simulink model "PlantArch"  (R2021b)
settings: Solver=VariableStepAuto  StartTime=0.0  StopTime=10.0  RelTol=1e-3
undefined symbols (not defined in the file or in its folder): N, P
libraries: nesl_utility x17, fl_lib x15, ee_lib x9
settings Model: DataDictionary=ZC_EVPowerSystem.sldd  Creator=ykamatan  LastModifiedBy=ykamatan

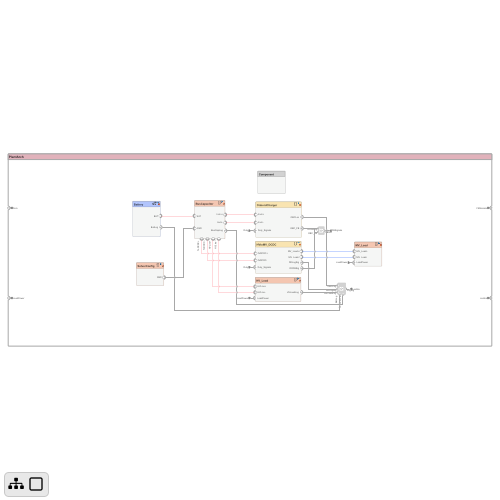
[thumbnail: Simulink's stored preview of the top-level diagram]
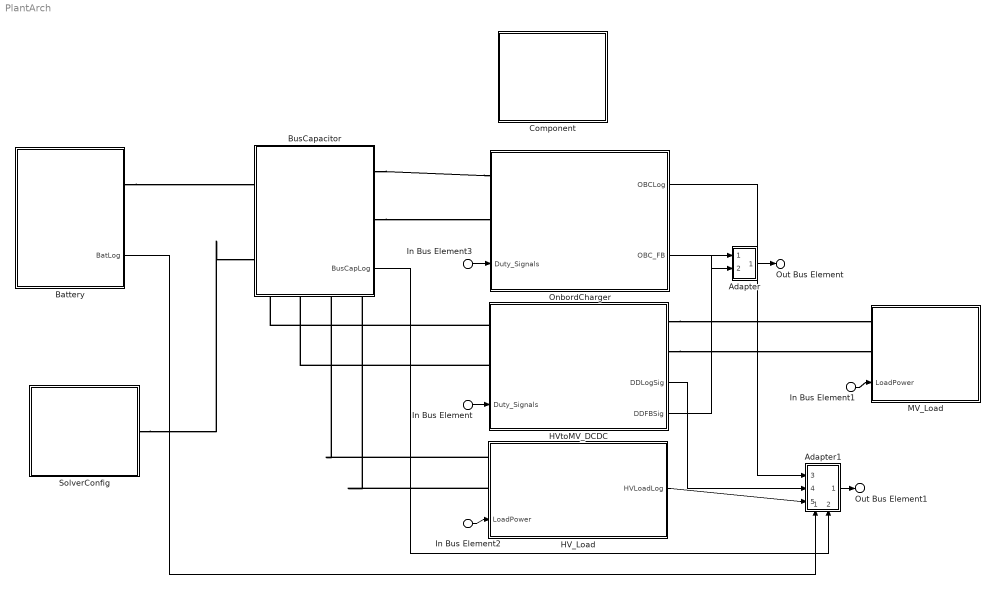
== system PlantArch ==
  In Bus Element : Inport  PortName=Duty
  In Bus Element3 : Inport  PortName=Duty
  In Bus Element1 : Inport  Port=2  PortName=LoadPower
  In Bus Element2 : Inport  Port=2  PortName=LoadPower
  Adapter : Subsystem
      settings: PortSchema="{\"entries\":[{\"content\":{\"margin\":10,\"minimumSpacing\":15,\"sides\":[{\"content\":{\"connectorIds\":[\"In1\",\"In2\"]},\"type\":\"ConnectorPlacement.EquallySpacedRectSide\",\"uuid\":\"68f5454e-c2f0-4736-99c3-02080df13840\"},{\"content\":{\"connectorIds\":[\"Out1\"],\"side\":\"RIGHT\"},\"type\":\"ConnectorPlacement.EquallySpacedRectSide\",\"uuid\":\"5ee879a6-3050-43f8-b648-386fe489b578\"},{\"content\":{\"connectorIds\":[],\"side\":\"TOP\"},\"type\":\"ConnectorPlacement.EquallySpacedRectSide\",\"uuid\":\"ef80faa4-f045-40f6-9eb7-7f3a67b10a8e\"}]},\"type\":\"ConnectorPlacement.EquallySpacedConnector\",\"uuid\":\"bb0e3b0d-aad0-4c98-a3b7-f5aab2b06e29\"}],\"packageUris\":[\"http://schema.mathworks.com/mf0/Connector/R2020b\"],\"version\":\"1.0\"}"
  Adapter1 : Subsystem
      settings: PortSchema="{\"entries\":[{\"content\":{\"margin\":10,\"minimumSpacing\":15,\"sides\":[{\"content\":{\"connectorIds\":[\"In3\",\"In4\",\"In5\"]},\"type\":\"ConnectorPlacement.EquallySpacedRectSide\",\"uuid\":\"68f5454e-c2f0-4736-99c3-02080df13840\"},{\"content\":{\"connectorIds\":[\"Out1\"],\"side\":\"RIGHT\"},\"type\":\"ConnectorPlacement.EquallySpacedRectSide\",\"uuid\":\"5ee879a6-3050-43f8-b648-386fe489b578\"},{\"content\":{\"connectorIds\":[],\"side\":\"TOP\"},\"type\":\"ConnectorPlacement.EquallySpacedRectSide\",\"uuid\":\"ef80faa4-f045-40f6-9eb7-7f3a67b10a8e\"},{\"content\":{\"connectorIds\":[\"In1\",\"In2\"],\"side\":\"BOTTOM\"},\"type\":\"ConnectorPlacement.EquallySpacedRectSide\",\"uuid\":\"e02d8c0b-11c6-4468-90e5-a6f684fa16b6\"}]},\"type\":\"ConnectorPlacement.EquallySpacedConnector\",\"uuid\":\"bb0e3b0d-aad0-4c98-a3b7-f5aab2b06e29\"}],\"packageUris\":[\"http://schema.mathworks.com/mf0/Connector/R2020b\"],\"version\":\"1.0\"}"
  Battery : Subsystem
      settings: PortSchema="{\"entries\":[{\"content\":{\"headerSize\":26,\"margin\":15,\"minimumSpacing\":25,\"sides\":[{\"content\":{\"connectorIds\":[]},\"type\":\"ConnectorPlacement.EquallySpacedRectSide\",\"uuid\":\"bc9bb9ba-2a95-4d32-9fa4-7976113ef647\"},{\"content\":{\"connectorIds\":[\"RConn1\",\"Out1\"],\"side\":\"RIGHT\"},\"type\":\"ConnectorPlacement.EquallySpacedRectSide\",\"uuid\":\"964ff6e2-b516-444b-80c9-2869b54c1800\"},{\"content\":{\"connectorIds\":[],\"side\":\"TOP\"},\"type\":\"ConnectorPlacement.EquallySpacedRectSide\",\"uuid\":\"d01200aa-db6c-474b-a6ec-1bd59e1bf90f\"}]},\"type\":\"ConnectorPlacement.EquallySpacedConnector\",\"uuid\":\"135e4cd7-10c4-47f4-80e9-6ecafc5508de\"}],\"packageUris\":[\"http://schema.mathworks.com/mf0/Connector/R2020b\"],\"version\":\"1.0\"}"
  BusCapacitor : Subsystem
      settings: PortSchema="{\"entries\":[{\"content\":{\"headerSize\":26,\"margin\":15,\"minimumSpacing\":25,\"sides\":[{\"content\":{\"connectorIds\":[\"LConn1\",\"LConn2\"]},\"type\":\"ConnectorPlacement.EquallySpacedRectSide\",\"uuid\":\"bc9bb9ba-2a95-4d32-9fa4-7976113ef647\"},{\"content\":{\"connectorIds\":[\"RConn5\",\"RConn6\",\"Out1\"],\"side\":\"RIGHT\"},\"type\":\"ConnectorPlacement.EquallySpacedRectSide\",\"uuid\":\"964ff6e2-b516-444b-80c9-2869b54c1800\"},{\"content\":{\"connectorIds\":[],\"side\":\"TOP\"},\"type\":\"ConnectorPlacement.EquallySpacedRectSide\",\"uuid\":\"d01200aa-db6c-474b-a6ec-1bd59e1bf90f\"},{\"content\":{\"connectorIds\":[\"RConn1\",\"RConn2\",\"RConn3\",\"RConn4\"],\"side\":\"BOTTOM\"},\"type\":\"ConnectorPlacement.EquallySpacedRectSide\",\"uuid\":\"7b919d1c-288c-41a8-8fd6-bd8ebd8eb2b7\"}]},\"type\":\"ConnectorPlacement.EquallySpacedConnector\",\"uuid\":\"135e4cd7-10c4-47f4-80e9-6ecafc5508de\"}],\"packageUris\":[\"http://schema.mathworks.com/mf0/Connector/R2020b\"],\"version\":\"1.0\"}"
  Component : Subsystem
      settings: PortSchema="{\"entries\":[{\"content\":{\"headerSize\":26,\"margin\":15,\"minimumSpacing\":25,\"sides\":[{\"content\":{\"connectorIds\":[]},\"type\":\"ConnectorPlacement.EquallySpacedRectSide\",\"uuid\":\"03ee5175-8d94-4deb-b18d-1b94bccaf658\"},{\"content\":{\"connectorIds\":[],\"side\":\"RIGHT\"},\"type\":\"ConnectorPlacement.EquallySpacedRectSide\",\"uuid\":\"44db8dae-2982-4fa1-b39b-413b881f7ee2\"},{\"content\":{\"connectorIds\":[],\"side\":\"TOP\"},\"type\":\"ConnectorPlacement.EquallySpacedRectSide\",\"uuid\":\"37e3387e-c8c6-4301-8ebe-99b8cda93072\"}]},\"type\":\"ConnectorPlacement.EquallySpacedConnector\",\"uuid\":\"c90e0097-298e-4f62-a136-d8f6219bd626\"}],\"packageUris\":[\"http://schema.mathworks.com/mf0/Connector/R2020b\"],\"version\":\"1.0\"}"
  HV_Load : Subsystem
      settings: PortSchema="{\"entries\":[{\"content\":{\"headerSize\":26,\"margin\":15,\"minimumSpacing\":25,\"sides\":[{\"content\":{\"connectorIds\":[\"LConn1\",\"LConn2\",\"In1\"]},\"type\":\"ConnectorPlacement.EquallySpacedRectSide\",\"uuid\":\"bc9bb9ba-2a95-4d32-9fa4-7976113ef647\"},{\"content\":{\"connectorIds\":[\"Out1\"],\"side\":\"RIGHT\"},\"type\":\"ConnectorPlacement.EquallySpacedRectSide\",\"uuid\":\"964ff6e2-b516-444b-80c9-2869b54c1800\"},{\"content\":{\"connectorIds\":[],\"side\":\"TOP\"},\"type\":\"ConnectorPlacement.EquallySpacedRectSide\",\"uuid\":\"d01200aa-db6c-474b-a6ec-1bd59e1bf90f\"}]},\"type\":\"ConnectorPlacement.EquallySpacedConnector\",\"uuid\":\"135e4cd7-10c4-47f4-80e9-6ecafc5508de\"}],\"packageUris\":[\"http://schema.mathworks.com/mf0/Connector/R2020b\"],\"version\":\"1.0\"}"
  HVtoMV_DCDC : Subsystem
      settings: PortSchema="{\"entries\":[{\"content\":{\"headerSize\":26,\"margin\":15,\"minimumSpacing\":25,\"sides\":[{\"content\":{\"connectorIds\":[\"LConn1\",\"LConn2\",\"In1\"]},\"type\":\"ConnectorPlacement.EquallySpacedRectSide\",\"uuid\":\"bc9bb9ba-2a95-4d32-9fa4-7976113ef647\"},{\"content\":{\"connectorIds\":[\"RConn1\",\"RConn2\",\"Out1\",\"Out2\"],\"side\":\"RIGHT\"},\"type\":\"ConnectorPlacement.EquallySpacedRectSide\",\"uuid\":\"964ff6e2-b516-444b-80c9-2869b54c1800\"},{\"content\":{\"connectorIds\":[],\"side\":\"TOP\"},\"type\":\"ConnectorPlacement.EquallySpacedRectSide\",\"uuid\":\"d01200aa-db6c-474b-a6ec-1bd59e1bf90f\"}]},\"type\":\"ConnectorPlacement.EquallySpacedConnector\",\"uuid\":\"135e4cd7-10c4-47f4-80e9-6ecafc5508de\"}],\"packageUris\":[\"http://schema.mathworks.com/mf0/Connector/R2020b\"],\"version\":\"1.0\"}"
  MV_Load : Subsystem
      settings: PortSchema="{\"entries\":[{\"content\":{\"headerSize\":26,\"margin\":15,\"minimumSpacing\":25,\"sides\":[{\"content\":{\"connectorIds\":[\"LConn1\",\"LConn2\",\"In1\"]},\"type\":\"ConnectorPlacement.EquallySpacedRectSide\",\"uuid\":\"bc9bb9ba-2a95-4d32-9fa4-7976113ef647\"},{\"content\":{\"connectorIds\":[],\"side\":\"RIGHT\"},\"type\":\"ConnectorPlacement.EquallySpacedRectSide\",\"uuid\":\"964ff6e2-b516-444b-80c9-2869b54c1800\"},{\"content\":{\"connectorIds\":[],\"side\":\"TOP\"},\"type\":\"ConnectorPlacement.EquallySpacedRectSide\",\"uuid\":\"d01200aa-db6c-474b-a6ec-1bd59e1bf90f\"}]},\"type\":\"ConnectorPlacement.EquallySpacedConnector\",\"uuid\":\"135e4cd7-10c4-47f4-80e9-6ecafc5508de\"}],\"packageUris\":[\"http://schema.mathworks.com/mf0/Connector/R2020b\"],\"version\":\"1.0\"}"
  OnbordCharger : Subsystem
      settings: PortSchema="{\"entries\":[{\"content\":{\"headerSize\":26,\"margin\":15,\"minimumSpacing\":25,\"sides\":[{\"content\":{\"connectorIds\":[\"LConn1\",\"LConn2\",\"In1\"]},\"type\":\"ConnectorPlacement.EquallySpacedRectSide\",\"uuid\":\"bc9bb9ba-2a95-4d32-9fa4-7976113ef647\"},{\"content\":{\"connectorIds\":[\"Out1\",\"Out2\"],\"side\":\"RIGHT\"},\"type\":\"ConnectorPlacement.EquallySpacedRectSide\",\"uuid\":\"964ff6e2-b516-444b-80c9-2869b54c1800\"},{\"content\":{\"connectorIds\":[],\"side\":\"TOP\"},\"type\":\"ConnectorPlacement.EquallySpacedRectSide\",\"uuid\":\"d01200aa-db6c-474b-a6ec-1bd59e1bf90f\"}]},\"type\":\"ConnectorPlacement.EquallySpacedConnector\",\"uuid\":\"135e4cd7-10c4-47f4-80e9-6ecafc5508de\"}],\"packageUris\":[\"http://schema.mathworks.com/mf0/Connector/R2020b\"],\"version\":\"1.0\"}"
  SolverConfig : Subsystem
      settings: PortSchema="{\"entries\":[{\"content\":{\"headerSize\":26,\"margin\":15,\"minimumSpacing\":25,\"sides\":[{\"content\":{\"connectorIds\":[]},\"type\":\"ConnectorPlacement.EquallySpacedRectSide\",\"uuid\":\"bc9bb9ba-2a95-4d32-9fa4-7976113ef647\"},{\"content\":{\"connectorIds\":[\"RConn1\"],\"side\":\"RIGHT\"},\"type\":\"ConnectorPlacement.EquallySpacedRectSide\",\"uuid\":\"964ff6e2-b516-444b-80c9-2869b54c1800\"},{\"content\":{\"connectorIds\":[],\"side\":\"TOP\"},\"type\":\"ConnectorPlacement.EquallySpacedRectSide\",\"uuid\":\"d01200aa-db6c-474b-a6ec-1bd59e1bf90f\"}]},\"type\":\"ConnectorPlacement.EquallySpacedConnector\",\"uuid\":\"135e4cd7-10c4-47f4-80e9-6ecafc5508de\"}],\"packageUris\":[\"http://schema.mathworks.com/mf0/Connector/R2020b\"],\"version\":\"1.0\"}"
  Out Bus Element : Outport  PortName=FBSignals
  Out Bus Element1 : Outport  Port=2  PortName=LogSig
  wires:
  In Bus Element1/1 -> MV_Load/1(LoadPower)
  In Bus Element/1 -> HVtoMV_DCDC/1(Duty_Signals)
  In Bus Element3/1 -> OnbordCharger/1(Duty_Signals)
  Adapter/1(FBSig) -> Out Bus Element/1
  Adapter1/1(LogSig) -> Out Bus Element1/1
  In Bus Element2/1 -> HV_Load/1(LoadPower)
  Battery/1(BatLog) -> Adapter1/1(BatLog)
  BusCapacitor/1(BusCapLog) -> Adapter1/2(BusCapLog)
  OnbordCharger/1(OBCLog) -> Adapter1/3(OBCLog)
  HVtoMV_DCDC/1(DDLogSig) -> Adapter1/4(DDLogSig)
  HV_Load/1(HVLoadLog) -> Adapter1/5(HVLoadLog)
  HVtoMV_DCDC/2(DDFBSig) -> Adapter/1(DDFBSig)
  OnbordCharger/2(OBC_FB) -> Adapter/2(OBC_FB)
  connections:
  HVtoMV_DCDC/RConn1 -- MV_Load/LConn1
  HVtoMV_DCDC/RConn2 -- MV_Load/LConn2
  HV_Load/LConn1 -- BusCapacitor/RConn3
  HV_Load/LConn2 -- BusCapacitor/RConn4
  HVtoMV_DCDC/LConn1 -- BusCapacitor/RConn1
  HVtoMV_DCDC/LConn2 -- BusCapacitor/RConn2
  BusCapacitor/RConn5 -- OnbordCharger/LConn1
  BusCapacitor/RConn6 -- OnbordCharger/LConn2
  SolverConfig/RConn1 -- BusCapacitor/LConn2
  Battery/RConn1 -- BusCapacitor/LConn1

== system PlantArch/Adapter ==
  Bus Element In2 : Inport  PortName=DDFBSig
  Bus Element In1 : Inport  Port=2  PortName=OBC_FB
  Out Bus Element : Outport  PortName=FBSig  Element=DD_FBSig
  BEP : Outport  PortName=FBSig  Element=PFC_FBSig
  wires:
  Bus Element In2/1 -> Out Bus Element/1
  Bus Element In1/1 -> BEP/1

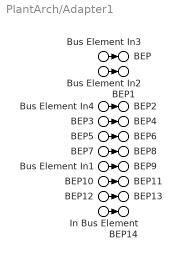
== system PlantArch/Adapter1 ==
  Bus Element In4 : Inport  PortName=BatLog  Element=iDC
  Bus Element In3 : Inport  Port=2  PortName=BusCapLog  Element=vDC
  Bus Element In2 : Inport  Port=3  PortName=OBCLog  Element=iL
  BEP3 : Inport  Port=3  PortName=OBCLog  Element=iDCInv
  BEP5 : Inport  Port=3  PortName=OBCLog  Element=vInv
  BEP7 : Inport  Port=3  PortName=OBCLog  Element=vs
  Bus Element In1 : Inport  Port=4  PortName=DDLogSig  Element=iLoad48V
  BEP10 : Inport  Port=4  PortName=DDLogSig  Element=iDC48VBass
  BEP12 : Inport  Port=4  PortName=DDLogSig  Element=v48VBass
  In Bus Element : Inport  Port=5  PortName=HVLoadLog  Element=iDC400VBass
  BEP1 : Outport  PortName=LogSig  Element=iL
  BEP2 : Outport  PortName=LogSig  Element=iDC
  BEP4 : Outport  PortName=LogSig  Element=iDCInv
  BEP9 : Outport  PortName=LogSig  Element=iLoad48V
  BEP11 : Outport  PortName=LogSig  Element=iDC48VBass
  BEP14 : Outport  PortName=LogSig  Element=iDC400VBass
  BEP : Outport  PortName=LogSig  Element=vDC
  BEP6 : Outport  PortName=LogSig  Element=vInv
  BEP8 : Outport  PortName=LogSig  Element=vs
  BEP13 : Outport  PortName=LogSig  Element=v48VBass
  wires:
  Bus Element In4/1 -> BEP2/1
  Bus Element In3/1 -> BEP/1
  Bus Element In2/1 -> BEP1/1
  BEP3/1 -> BEP4/1
  BEP5/1 -> BEP6/1
  BEP7/1 -> BEP8/1
  Bus Element In1/1 -> BEP9/1
  BEP10/1 -> BEP11/1
  BEP12/1 -> BEP13/1
  In Bus Element/1 -> BEP14/1

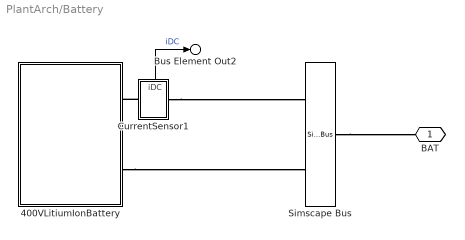
== system PlantArch/Battery ==
  400VLitiumIonBattery : Subsystem
  CurrentSensor1 : Subsystem
      settings: PortSchema="{\"entries\":[{\"content\":{\"sides\":[{\"content\":{\"connectorIds\":[\"LConn1\"]},\"type\":\"ConnectorPlacement.EquallySpacedRectSide\",\"uuid\":\"7286f59e-cee0-499d-832c-cf6f33a1b017\"},{\"content\":{\"connectorIds\":[\"RConn1\"],\"side\":\"RIGHT\"},\"type\":\"ConnectorPlacement.EquallySpacedRectSide\",\"uuid\":\"6a983281-a6bc-4a57-a5ba-c4da9a8828f4\"},{\"content\":{\"connectorIds\":[\"Out1\"],\"side\":\"TOP\"},\"type\":\"ConnectorPlacement.EquallySpacedRectSide\",\"uuid\":\"6969f7e7-2dce-4d64-b6f6-e92ef9035b1a\"}]},\"type\":\"ConnectorPlacement.EquallySpacedConnector\",\"uuid\":\"05fc616a-5402-4b75-b59e-8cf259d71f3d\"}],\"packageUris\":[\"http://schema.mathworks.com/mf0/Connector/R2020b\"],\"version\":\"1.0\"}"
  Simscape Bus : SimscapeBus  HierarchyStrings=P;N  ConnectionType=Bus: HV_PowerLine
  BAT : PMIOPort  Side=Right  ConnectionType=Bus: HV_PowerLine
  Bus Element Out2 : Outport  PortName=BatLog  Element=iDC
  wires:
  CurrentSensor1/1(iDC) -> Bus Element Out2/1  "iDC"
  connections:
  CurrentSensor1/LConn1 -- 400VLitiumIonBattery/RConn1
  CurrentSensor1/RConn1 -- Simscape Bus/LConn1
  400VLitiumIonBattery/RConn2 -- Simscape Bus/LConn2
  Simscape Bus/RConn1 -- BAT/RConn1

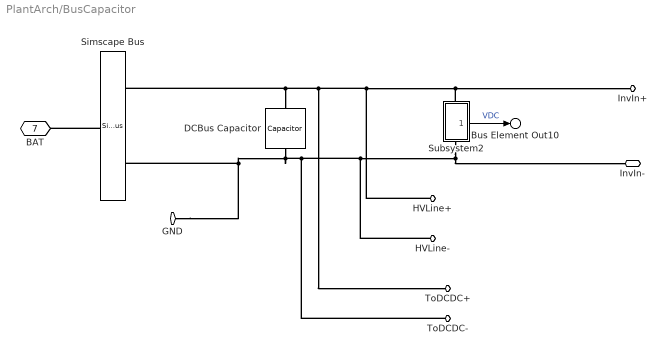
== system PlantArch/BusCapacitor ==
  DCBus Capacitor : ee_lib/Passive/Capacitor  cap_option=0  c=1000e-6 F  Cvec=[1e-05, 1e-06] F  Vvec=[0, 10] V  CV_table_symmetry=1  f_vec=[1, 10] kHz  DFext_vec=[.8, 1.2]  C_tol=5  enable_C_tol=0  tol_distribution=1  nSigma=4  r=1e-6 Ohm  g=0 1/Ohm  averaging_period=0 s  enable_operating_limits=0  operating_limit_action=2  max_working_voltage_range=[-25, 25] V  power_rating=1 W  enable_faults=0  fault_action=1  Cscale_faulted=100  R_faulted=1e-3 Ohm  G_faulted=0 1/Ohm  tau_fault=1e-3 s  enable_temporal_fault=0  t_fault=1 s  enable_behavioral_fault=0  max_permissible_voltage_range=[-100, 100] V  t_fail_on_voltage=1 s  i_specify=off  i_priority=None  i=0 A  i_nominal_specify=off  i_nominal_unit=A  i_nominal_value=1  v_specify=off  v_priority=None  v=400 V  v_nominal_specify=off  v_nominal_unit=V  v_nominal_value=1  vc_specify=on  vc_priority=High  vc=400 V  vc_nominal_specify=off  vc_nominal_unit=V  vc_nominal_value=1
  Simscape Bus : SimscapeBus  HierarchyStrings=P;N  ConnectionType=Bus: HV_PowerLine
  Subsystem2 : Subsystem
      settings: PortSchema="{\"entries\":[{\"content\":{\"sides\":[{\"content\":{\"connectorIds\":[]},\"type\":\"ConnectorPlacement.EquallySpacedRectSide\",\"uuid\":\"7286f59e-cee0-499d-832c-cf6f33a1b017\"},{\"content\":{\"connectorIds\":[\"Out1\"],\"side\":\"RIGHT\"},\"type\":\"ConnectorPlacement.EquallySpacedRectSide\",\"uuid\":\"6a983281-a6bc-4a57-a5ba-c4da9a8828f4\"},{\"content\":{\"connectorIds\":[\"LConn1\"],\"side\":\"TOP\"},\"type\":\"ConnectorPlacement.EquallySpacedRectSide\",\"uuid\":\"6969f7e7-2dce-4d64-b6f6-e92ef9035b1a\"},{\"content\":{\"connectorIds\":[\"RConn1\"],\"side\":\"BOTTOM\"},\"type\":\"ConnectorPlacement.EquallySpacedRectSide\",\"uuid\":\"8f7d22cd-967a-487e-912d-7270502758f1\"}]},\"type\":\"ConnectorPlacement.EquallySpacedConnector\",\"uuid\":\"05fc616a-5402-4b75-b59e-8cf259d71f3d\"}],\"packageUris\":[\"http://schema.mathworks.com/mf0/Connector/R2020b\"],\"version\":\"1.0\"}"
  ToDCDC+ : PMIOPort  Side=Right
  ToDCDC- : PMIOPort  Port=2  Side=Right
  HVLine+ : PMIOPort  Port=3  Side=Right
  HVLine- : PMIOPort  Port=4  Side=Right
  InvIn+ : PMIOPort  Port=5  Side=Right
  InvIn- : PMIOPort  Port=6  Side=Right
  BAT : PMIOPort  Port=7  Side=Left  ConnectionType=Bus: HV_PowerLine
  GND : PMIOPort  Port=8  Side=Left
  Bus Element Out10 : Outport  PortName=BusCapLog  Element=vDC
  wires:
  Subsystem2/1(Vdc) -> Bus Element Out10/1  "VDC"
  connections:
  DCBus Capacitor/RConn1 -- GND/RConn1 -- Simscape Bus/LConn2 -- HVLine-/RConn1 -- InvIn-/RConn1 -- Subsystem2/RConn1 -- ToDCDC-/RConn1
  HVLine+/RConn1 -- InvIn+/RConn1 -- Subsystem2/LConn1 -- ToDCDC+/RConn1 -- DCBus Capacitor/LConn1 -- Simscape Bus/LConn1
  Simscape Bus/RConn1 -- BAT/RConn1

== system PlantArch/Component ==

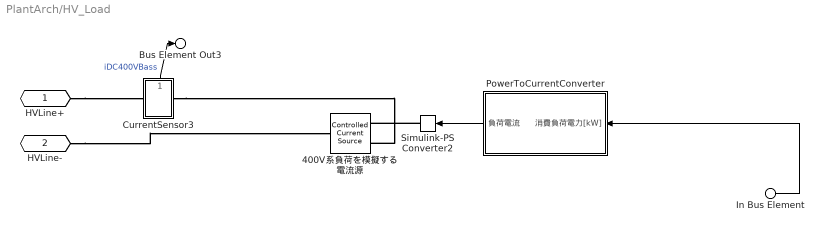
== system PlantArch/HV_Load ==
  In Bus Element : Inport  PortName=LoadPower  Element=Load400V
  400V系負荷を模擬する 電流源 : fl_lib/Electrical/Electrical Sources/Controlled Current Source
  CurrentSensor3 : Subsystem
      settings: PortSchema="{\"entries\":[{\"content\":{\"sides\":[{\"content\":{\"connectorIds\":[\"LConn1\"]},\"type\":\"ConnectorPlacement.EquallySpacedRectSide\",\"uuid\":\"7286f59e-cee0-499d-832c-cf6f33a1b017\"},{\"content\":{\"connectorIds\":[\"RConn1\"],\"side\":\"RIGHT\"},\"type\":\"ConnectorPlacement.EquallySpacedRectSide\",\"uuid\":\"6a983281-a6bc-4a57-a5ba-c4da9a8828f4\"},{\"content\":{\"connectorIds\":[\"Out1\"],\"side\":\"TOP\"},\"type\":\"ConnectorPlacement.EquallySpacedRectSide\",\"uuid\":\"6969f7e7-2dce-4d64-b6f6-e92ef9035b1a\"}]},\"type\":\"ConnectorPlacement.EquallySpacedConnector\",\"uuid\":\"05fc616a-5402-4b75-b59e-8cf259d71f3d\"}],\"packageUris\":[\"http://schema.mathworks.com/mf0/Connector/R2020b\"],\"version\":\"1.0\"}"
  PowerToCurrentConverter : Subsystem
  Simulink-PS Converter2 : nesl_utility/Simulink-PS Converter  PhysicalDomain=network_engine_domain  SubClassName=ps_input  LeftPortType=input  RightPortType=output  PseudoPeriodic=off  Frequencies=[]  NoiseDistribution=none  NoiseParameters=[]  Unit=1  AffineConversion=off  FilteringAndDerivatives=provide  SimscapeFilterOrder=1  InputFilterTimeConstant=0.001  UdotUserProvided=0
      settings: SourceProductBaseCode=PW,SS
  HVLine+ : PMIOPort  Side=Left
  HVLine- : PMIOPort  Port=2  Side=Left
  Bus Element Out3 : Outport  PortName=HVLoadLog  Element=iDC400VBass
  wires:
  CurrentSensor3/1(iDC400VBass) -> Bus Element Out3/1  "iDC400VBass"
  PowerToCurrentConverter/1(負荷電流) -> Simulink-PS Converter2/1
  In Bus Element/1 -> PowerToCurrentConverter/1(消費負荷電力[kW])
  connections:
  Simulink-PS Converter2/RConn1 -- 400V系負荷を模擬する 電流源/RConn1
  CurrentSensor3/RConn1 -- 400V系負荷を模擬する 電流源/RConn2
  HVLine+/RConn1 -- CurrentSensor3/LConn1
  HVLine-/RConn1 -- 400V系負荷を模擬する 電流源/LConn1

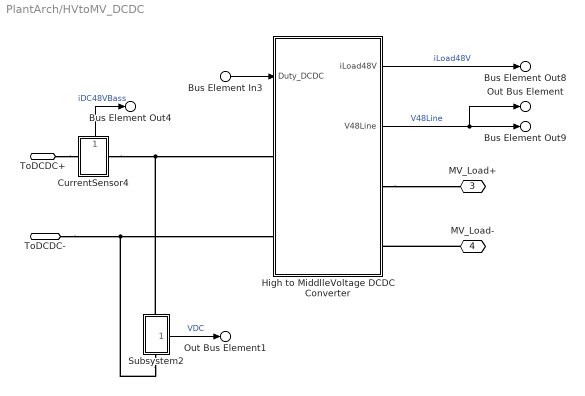
== system PlantArch/HVtoMV_DCDC ==
  Bus Element In3 : Inport  PortName=Duty_Signals  Element=DD48v_Duty
  CurrentSensor4 : Subsystem
      settings: PortSchema="{\"entries\":[{\"content\":{\"sides\":[{\"content\":{\"connectorIds\":[\"LConn1\"]},\"type\":\"ConnectorPlacement.EquallySpacedRectSide\",\"uuid\":\"7286f59e-cee0-499d-832c-cf6f33a1b017\"},{\"content\":{\"connectorIds\":[\"RConn1\"],\"side\":\"RIGHT\"},\"type\":\"ConnectorPlacement.EquallySpacedRectSide\",\"uuid\":\"6a983281-a6bc-4a57-a5ba-c4da9a8828f4\"},{\"content\":{\"connectorIds\":[\"Out1\"],\"side\":\"TOP\"},\"type\":\"ConnectorPlacement.EquallySpacedRectSide\",\"uuid\":\"6969f7e7-2dce-4d64-b6f6-e92ef9035b1a\"}]},\"type\":\"ConnectorPlacement.EquallySpacedConnector\",\"uuid\":\"05fc616a-5402-4b75-b59e-8cf259d71f3d\"}],\"packageUris\":[\"http://schema.mathworks.com/mf0/Connector/R2020b\"],\"version\":\"1.0\"}"
  High to MiddlleVoltage DCDC Converter : Subsystem
  Subsystem2 : Subsystem
      settings: PortSchema="{\"entries\":[{\"content\":{\"sides\":[{\"content\":{\"connectorIds\":[]},\"type\":\"ConnectorPlacement.EquallySpacedRectSide\",\"uuid\":\"7286f59e-cee0-499d-832c-cf6f33a1b017\"},{\"content\":{\"connectorIds\":[\"Out1\"],\"side\":\"RIGHT\"},\"type\":\"ConnectorPlacement.EquallySpacedRectSide\",\"uuid\":\"6a983281-a6bc-4a57-a5ba-c4da9a8828f4\"},{\"content\":{\"connectorIds\":[\"LConn1\"],\"side\":\"TOP\"},\"type\":\"ConnectorPlacement.EquallySpacedRectSide\",\"uuid\":\"6969f7e7-2dce-4d64-b6f6-e92ef9035b1a\"},{\"content\":{\"connectorIds\":[\"RConn1\"],\"side\":\"BOTTOM\"},\"type\":\"ConnectorPlacement.EquallySpacedRectSide\",\"uuid\":\"8f7d22cd-967a-487e-912d-7270502758f1\"}]},\"type\":\"ConnectorPlacement.EquallySpacedConnector\",\"uuid\":\"05fc616a-5402-4b75-b59e-8cf259d71f3d\"}],\"packageUris\":[\"http://schema.mathworks.com/mf0/Connector/R2020b\"],\"version\":\"1.0\"}"
  ToDCDC+ : PMIOPort  Side=Left
  ToDCDC- : PMIOPort  Port=2  Side=Left
  MV_Load+ : PMIOPort  Port=3  Side=Right
  MV_Load- : PMIOPort  Port=4  Side=Right
  Bus Element Out8 : Outport  PortName=DDLogSig  Element=iLoad48V
  Bus Element Out4 : Outport  PortName=DDLogSig  Element=iDC48VBass
  Bus Element Out9 : Outport  PortName=DDLogSig  Element=v48VBass
  Out Bus Element : Outport  Port=2  PortName=DDFBSig  Element=vout
  Out Bus Element1 : Outport  Port=2  PortName=DDFBSig  Element=vin
  wires:
  CurrentSensor4/1(iDC48VBass) -> Bus Element Out4/1  "iDC48VBass"
  Bus Element In3/1 -> High to MiddlleVoltage DCDC Converter/1(Duty_DCDC)
  High to MiddlleVoltage DCDC Converter/2(V48Line) -> Out Bus Element/1, Bus Element Out9/1  "V48Line"
  High to MiddlleVoltage DCDC Converter/1(iLoad48V) -> Bus Element Out8/1  "iLoad48V"
  Subsystem2/1(Vdc) -> Out Bus Element1/1  "VDC"
  connections:
  CurrentSensor4/RConn1 -- Subsystem2/LConn1 -- High to MiddlleVoltage DCDC Converter/LConn1
  High to MiddlleVoltage DCDC Converter/RConn1 -- MV_Load+/RConn1
  MV_Load-/RConn1 -- High to MiddlleVoltage DCDC Converter/RConn2
  ToDCDC+/RConn1 -- CurrentSensor4/LConn1
  ToDCDC-/RConn1 -- Subsystem2/RConn1 -- High to MiddlleVoltage DCDC Converter/LConn2

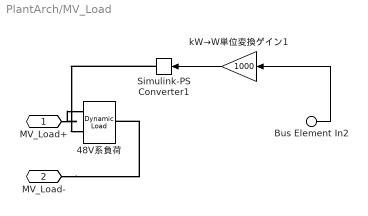
== system PlantArch/MV_Load ==
  Bus Element In2 : Inport  PortName=LoadPower  Element=Load48V
  48V系負荷 : ee_lib/Passive/Dynamic Load  load_type=ee.enum.dc_ac.dc  min_supply_voltage=38 V  pow_min=1e-3 W  G_reverse=1e-6 S  deltaV=1e-3 V  f0=60 Hz  Vrms_min=200 V  Pmin=1e-3 W  enable_fault=simscape.enum.onoff.off  fault_action=simscape.enum.assert.action.none  t_fault=1 s  open_conductance=1e-4 S
      settings: SourceProductBaseCode=PS  InternalSimscapePortConfiguration="{\"Bottom\":[],\"Left\":[{\"id\":\"p\",\"label\":\"+\",\"type\":\"foundation.electrical.electrical\"}],\"Right\":[{\"id\":\"n\",\"label\":\"-\",\"type\":\"foundation.electrical.electrical\"}],\"Top\":[{\"id\":\"P\",\"label\":\"P\",\"type\":\"input\"}]}"
  Simulink-PS Converter1 : nesl_utility/Simulink-PS Converter  PhysicalDomain=network_engine_domain  SubClassName=ps_input  LeftPortType=input  RightPortType=output  PseudoPeriodic=off  Frequencies=[]  NoiseDistribution=none  NoiseParameters=[]  Unit=1  AffineConversion=off  FilteringAndDerivatives=provide  SimscapeFilterOrder=1  InputFilterTimeConstant=0.001  UdotUserProvided=0
      settings: SourceProductBaseCode=PW,SS
  kW→W単位変換ゲイン1 : Gain  Gain=1000
  MV_Load+ : PMIOPort  Side=Left
  MV_Load- : PMIOPort  Port=2  Side=Left
  wires:
  kW→W単位変換ゲイン1/1 -> Simulink-PS Converter1/1
  Bus Element In2/1 -> kW→W単位変換ゲイン1/1
  connections:
  Simulink-PS Converter1/RConn1 -- 48V系負荷/LConn2
  MV_Load-/RConn1 -- 48V系負荷/RConn1
  MV_Load+/RConn1 -- 48V系負荷/LConn1

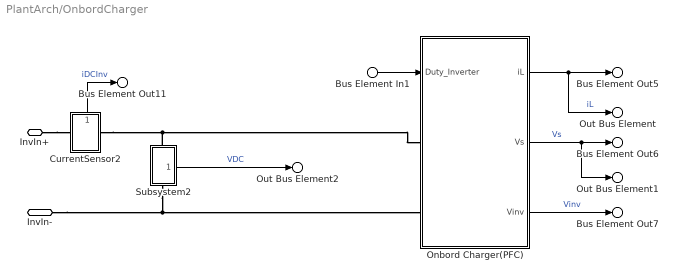
== system PlantArch/OnbordCharger ==
  Bus Element In1 : Inport  PortName=Duty_Signals  Element=PFC_Duty
  CurrentSensor2 : Subsystem
      settings: PortSchema="{\"entries\":[{\"content\":{\"sides\":[{\"content\":{\"connectorIds\":[\"LConn1\"]},\"type\":\"ConnectorPlacement.EquallySpacedRectSide\",\"uuid\":\"7286f59e-cee0-499d-832c-cf6f33a1b017\"},{\"content\":{\"connectorIds\":[\"RConn1\"],\"side\":\"RIGHT\"},\"type\":\"ConnectorPlacement.EquallySpacedRectSide\",\"uuid\":\"6a983281-a6bc-4a57-a5ba-c4da9a8828f4\"},{\"content\":{\"connectorIds\":[\"Out1\"],\"side\":\"TOP\"},\"type\":\"ConnectorPlacement.EquallySpacedRectSide\",\"uuid\":\"6969f7e7-2dce-4d64-b6f6-e92ef9035b1a\"}]},\"type\":\"ConnectorPlacement.EquallySpacedConnector\",\"uuid\":\"05fc616a-5402-4b75-b59e-8cf259d71f3d\"}],\"packageUris\":[\"http://schema.mathworks.com/mf0/Connector/R2020b\"],\"version\":\"1.0\"}"
  Onbord Charger(PFC) : Subsystem
  Subsystem2 : Subsystem
      settings: PortSchema="{\"entries\":[{\"content\":{\"sides\":[{\"content\":{\"connectorIds\":[]},\"type\":\"ConnectorPlacement.EquallySpacedRectSide\",\"uuid\":\"7286f59e-cee0-499d-832c-cf6f33a1b017\"},{\"content\":{\"connectorIds\":[\"Out1\"],\"side\":\"RIGHT\"},\"type\":\"ConnectorPlacement.EquallySpacedRectSide\",\"uuid\":\"6a983281-a6bc-4a57-a5ba-c4da9a8828f4\"},{\"content\":{\"connectorIds\":[\"LConn1\"],\"side\":\"TOP\"},\"type\":\"ConnectorPlacement.EquallySpacedRectSide\",\"uuid\":\"6969f7e7-2dce-4d64-b6f6-e92ef9035b1a\"},{\"content\":{\"connectorIds\":[\"RConn1\"],\"side\":\"BOTTOM\"},\"type\":\"ConnectorPlacement.EquallySpacedRectSide\",\"uuid\":\"8f7d22cd-967a-487e-912d-7270502758f1\"}]},\"type\":\"ConnectorPlacement.EquallySpacedConnector\",\"uuid\":\"05fc616a-5402-4b75-b59e-8cf259d71f3d\"}],\"packageUris\":[\"http://schema.mathworks.com/mf0/Connector/R2020b\"],\"version\":\"1.0\"}"
  InvIn+ : PMIOPort  Side=Left
  InvIn- : PMIOPort  Port=2  Side=Left
  Bus Element Out5 : Outport  PortName=OBCLog  Element=iL
  Bus Element Out11 : Outport  PortName=OBCLog  Element=iDCInv
  Bus Element Out7 : Outport  PortName=OBCLog  Element=vInv
  Bus Element Out6 : Outport  PortName=OBCLog  Element=vs
  Out Bus Element1 : Outport  Port=2  PortName=OBC_FB  Element=vs
  Out Bus Element2 : Outport  Port=2  PortName=OBC_FB  Element=vdc
  Out Bus Element : Outport  Port=2  PortName=OBC_FB  Element=iL
  wires:
  Onbord Charger(PFC)/2(Vs) -> Out Bus Element1/1, Bus Element Out6/1  "Vs"
  Onbord Charger(PFC)/3(Vinv) -> Bus Element Out7/1  "Vinv"
  Onbord Charger(PFC)/1(iL) -> Out Bus Element/1, Bus Element Out5/1  "iL"
  Bus Element In1/1 -> Onbord Charger(PFC)/1(Duty_Inverter)
  CurrentSensor2/1(iDCInv) -> Bus Element Out11/1  "iDCInv"
  Subsystem2/1(Vdc) -> Out Bus Element2/1  "VDC"
  connections:
  CurrentSensor2/RConn1 -- Subsystem2/LConn1 -- Onbord Charger(PFC)/LConn1
  InvIn-/RConn1 -- Subsystem2/RConn1 -- Onbord Charger(PFC)/LConn2
  InvIn+/RConn1 -- CurrentSensor2/LConn1

== system PlantArch/SolverConfig ==
  Electrical Reference : fl_lib/Electrical/Electrical Elements/Electrical Reference
  Solver Configuration : nesl_utility/Solver Configuration  PhysicalDomain=network_engine_domain  SubClassName=solver  LeftPortType=input  RightPortType=generic  Tones=[]  Harmonics=[]  SimulateNoise=off  Profile=off  UseLocalSampling=off  EnableSwitchedLinearOptims=on  FrequencyDomain=off  UseCCode=off  RelTol=0.001  AbsTol=1e-06  MinStep=1e-09  ToWorkspace=off  RevertToSquareIcSolve=off  NumHomotopyIterations=100  PhasorMode=off  PhasorModeNumHarmonics=1  DoDC=off  ResidualTolerance=1e-09  UseLocalSolver=off  LocalSolverChoice=NE_BACKWARD_EULER_ADVANCER  LocalSolverSampleTime=0.001  DoFixedCost=off  MaxNonlinIter=3  MaxModeIter=2  ComputeImpulses=off  ImpulseIterations=2  LinearAlgebra=auto  EquationFormulation=NE_TIME_EF  DelaysMemoryBudget=1024  AutomaticFiltering=on  FilteringTimeConstant=0.001  PartitionStorageMethod=AS_NEEDED  PartitionMemoryBudget=1024  PartitionMethod=ROBUST
      settings: SourceProductBaseCode=PW,SS
  GND : PMIOPort  Side=Right
  connections:
  Electrical Reference/LConn1 -- GND/RConn1 -- Solver Configuration/RConn1

== system PlantArch/Battery/400VLitiumIonBattery ==
  400V 理想特性蓄電池 : ee_lib/Sources/Battery  Vnom=400 V  prm_dir=1  R1_dis=2 Ohm  R1_ch=2 Ohm  R1=1 Ohm  prm_AH=2  AH=0.5 hr*A  V1=380 V  AH1=0.25 hr*A  prm_R2=1  R2=2000 Ohm  prm_dyn=2  Rp1=0.05 Ohm  tau1=30 s  Rp2=0.005 Ohm  tau2=30 s  Rp3=0.005 Ohm  tau3=30 s  Rp4=0.005 Ohm  tau4=30 s  Rp5=0.005 Ohm  tau5=30 s  prm_fade=1  N_fade=100  AH_fade=45 hr*A  R1_fade=2.02 Ohm  R1_ch_fade=2.02 Ohm  V1_fade=10.35 V  prm_age=1  prm_age_OCV=1  OCV_age=0.9  SOC_age=60  delta_time_age_vec=[0] d  temperature_age_vec=[273] K  OCV_scaling_age=2.2134e6  OCV_offset_age=1.632e6  temp_exp_age=0.515833569 V  t_exp_age=0.75  i_specify=off  i_priority=None  i=0 A  i_nominal_specify=off  i_nominal_unit=A  i_nominal_value=1  v_specify=off  v_priority=None  v=0 V  v_nominal_specify=off  v_nominal_unit=V  v_nominal_value=1  charge_specify=on  charge_priority=High  charge=0.25 hr*A  charge_nominal_specify=off  charge_nominal_unit=hr*A  charge_nominal_value=1  num_cycles_specify=off  num_cycles_priority=High  num_cycles=0  num_cycles_nominal_specify=off  num_cycles_nominal_unit=1  num_cycles_nominal_value=1  Tmeas=298.15 K  Tmeas_age=298.15 K  Vnom_T2=12 V  R1_T2=2.2 Ohm  R1_T2_dis=2.2 Ohm  R1_T2_ch=2.2 Ohm  V1_T2=11.4 V  R2_T2=2200 Ohm  Rp1_T2=0.005 Ohm  tau1_T2=30 s  Rp2_T2=0.005 Ohm  tau2_T2=30 s  Rp3_T2=0.005 Ohm  tau3_T2=30 s  Rp4_T2=0.005 Ohm  tau4_T2=30 s  Rp5_T2=0.005 Ohm  tau5_T2=30 s  Tmeas2=273.15 K  thermal_mass=30000 J/K  temperature_specify=off  temperature_priority=High  temperature=298.15 K  temperature_nominal_specify=off  temperature_nominal_unit=K  temperature_nominal_value=1
  Bat+ : PMIOPort  Side=Right
  Bat- : PMIOPort  Port=2  Side=Right
  connections:
  400V 理想特性蓄電池/RConn1 -- Bat-/RConn1
  Bat+/RConn1 -- 400V 理想特性蓄電池/LConn1

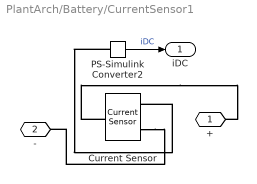
== system PlantArch/Battery/CurrentSensor1 ==
  Current Sensor : fl_lib/Electrical/Electrical Sensors/Current Sensor
  PS-Simulink Converter2 : nesl_utility/PS-Simulink Converter  PhysicalDomain=network_engine_domain  SubClassName=ps_output  LeftPortType=input  RightPortType=output  PseudoPeriodic=off  Frequencies=[]  Unit=inherit  AffineConversion=off
      settings: SourceProductBaseCode=PW,SS
  + : PMIOPort  Side=Left
  - : PMIOPort  Port=2  Side=Right
  iDC : Outport
  wires:
  PS-Simulink Converter2/1 -> iDC/1  "iDC"
  connections:
  Current Sensor/RConn2 -- -/RConn1
  PS-Simulink Converter2/LConn1 -- Current Sensor/RConn1
  Current Sensor/LConn1 -- +/RConn1

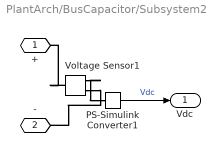
== system PlantArch/BusCapacitor/Subsystem2 ==
  PS-Simulink Converter1 : nesl_utility/PS-Simulink Converter  PhysicalDomain=network_engine_domain  SubClassName=ps_output  LeftPortType=input  RightPortType=output  PseudoPeriodic=off  Frequencies=[]  Unit=inherit  AffineConversion=off
      settings: SourceProductBaseCode=PW,SS
  Voltage Sensor1 : fl_lib/Electrical/Electrical Sensors/Voltage Sensor
  + : PMIOPort  Side=Left
  - : PMIOPort  Port=2  Side=Right
  Vdc : Outport
  wires:
  PS-Simulink Converter1/1 -> Vdc/1  "Vdc"
  connections:
  Voltage Sensor1/RConn2 -- -/RConn1
  Voltage Sensor1/LConn1 -- +/RConn1
  Voltage Sensor1/RConn1 -- PS-Simulink Converter1/LConn1

== system PlantArch/HV_Load/CurrentSensor3 ==
  Current Sensor : fl_lib/Electrical/Electrical Sensors/Current Sensor
  PS-Simulink Converter2 : nesl_utility/PS-Simulink Converter  PhysicalDomain=network_engine_domain  SubClassName=ps_output  LeftPortType=input  RightPortType=output  PseudoPeriodic=off  Frequencies=[]  Unit=inherit  AffineConversion=off
      settings: SourceProductBaseCode=PW,SS
  + : PMIOPort  Side=Left
  - : PMIOPort  Port=2  Side=Right
  iDC400VBass : Outport
  wires:
  PS-Simulink Converter2/1 -> iDC400VBass/1  "iDC400VBass"
  connections:
  Current Sensor/RConn2 -- -/RConn1
  PS-Simulink Converter2/LConn1 -- Current Sensor/RConn1
  Current Sensor/LConn1 -- +/RConn1

== system PlantArch/HV_Load/PowerToCurrentConverter ==
  消費負荷電力[kW] : Inport
  Divide : Product  Inputs=*/
  VDC_Typ値 : Constant  Value=400
  kW→W単位変換ゲイン : Gain  Gain=1000
  負荷電流 : Outport
  wires:
  Divide/1 -> 負荷電流/1
  VDC_Typ値/1 -> Divide/2
  kW→W単位変換ゲイン/1 -> Divide/1
  消費負荷電力[kW]/1 -> kW→W単位変換ゲイン/1

== system PlantArch/HVtoMV_DCDC/CurrentSensor4 ==
  Current Sensor : fl_lib/Electrical/Electrical Sensors/Current Sensor
  PS-Simulink Converter2 : nesl_utility/PS-Simulink Converter  PhysicalDomain=network_engine_domain  SubClassName=ps_output  LeftPortType=input  RightPortType=output  PseudoPeriodic=off  Frequencies=[]  Unit=inherit  AffineConversion=off
      settings: SourceProductBaseCode=PW,SS
  + : PMIOPort  Side=Left
  - : PMIOPort  Port=2  Side=Right
  iDC48VBass : Outport
  wires:
  PS-Simulink Converter2/1 -> iDC48VBass/1  "iDC48VBass"
  connections:
  Current Sensor/RConn2 -- -/RConn1
  PS-Simulink Converter2/LConn1 -- Current Sensor/RConn1
  Current Sensor/LConn1 -- +/RConn1

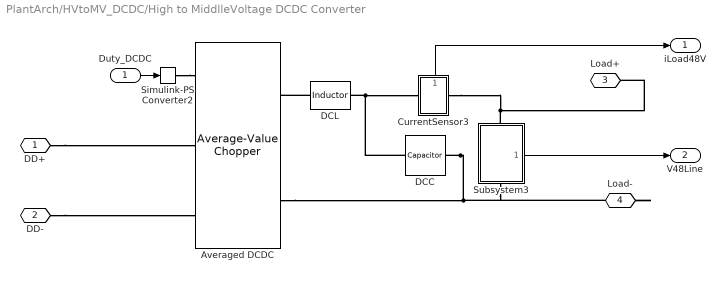
== system PlantArch/HVtoMV_DCDC/High to MiddlleVoltage DCDC Converter ==
  Duty_DCDC : Inport
  Averaged DCDC : ee_lib/Semiconductors & Converters/Converters/Average-Value Chopper  chopper_type=5  efficiency_option=1  efficiency_fixed=100  i_vec=[0, 2, 5] A  efficiency_vec=[90, 95, 98]
      settings: SourceProductBaseCode=PS  InternalSimscapePortConfiguration="{\"Bottom\":[],\"Left\":[{\"id\":\"DutyCycle\",\"label\":\"DutyCycle\",\"type\":\"input\"},{\"id\":\"p1\",\"label\":\"1+\",\"type\":\"foundation.electrical.electrical\"},{\"id\":\"n1\",\"label\":\"1-\",\"type\":\"foundation.electrical.electrical\"}],\"Right\":[{\"id\":\"p2\",\"label\":\"2+\",\"type\":\"foundation.electrical.electrical\"},{\"id\":\"n2\",\"label\":\"2-\",\"type\":\"foundation.electrical.electrical\"}],\"Top\":[]}"
  CurrentSensor3 : Subsystem
      settings: PortSchema="{\"entries\":[{\"content\":{\"sides\":[{\"content\":{\"connectorIds\":[\"LConn1\"]},\"type\":\"ConnectorPlacement.EquallySpacedRectSide\",\"uuid\":\"7286f59e-cee0-499d-832c-cf6f33a1b017\"},{\"content\":{\"connectorIds\":[\"RConn1\"],\"side\":\"RIGHT\"},\"type\":\"ConnectorPlacement.EquallySpacedRectSide\",\"uuid\":\"6a983281-a6bc-4a57-a5ba-c4da9a8828f4\"},{\"content\":{\"connectorIds\":[\"Out1\"],\"side\":\"TOP\"},\"type\":\"ConnectorPlacement.EquallySpacedRectSide\",\"uuid\":\"6969f7e7-2dce-4d64-b6f6-e92ef9035b1a\"}]},\"type\":\"ConnectorPlacement.EquallySpacedConnector\",\"uuid\":\"05fc616a-5402-4b75-b59e-8cf259d71f3d\"}],\"packageUris\":[\"http://schema.mathworks.com/mf0/Connector/R2020b\"],\"version\":\"1.0\"}"
  DCC : ee_lib/Passive/Capacitor  cap_option=0  c=100e-6 F  Cvec=[1e-05, 1e-06] F  Vvec=[0, 10] V  CV_table_symmetry=1  f_vec=[1, 10] kHz  DFext_vec=[.8, 1.2]  C_tol=5  enable_C_tol=0  tol_distribution=1  nSigma=4  r=100e-3 Ohm  g=0 1/Ohm  averaging_period=0 s  enable_operating_limits=0  operating_limit_action=2  max_working_voltage_range=[-25, 25] V  power_rating=1 W  enable_faults=0  fault_action=1  Cscale_faulted=100  R_faulted=1e-3 Ohm  G_faulted=0 1/Ohm  tau_fault=1e-3 s  enable_temporal_fault=0  t_fault=1 s  enable_behavioral_fault=0  max_permissible_voltage_range=[-100, 100] V  t_fail_on_voltage=1 s  i_specify=off  i_priority=None  i=0 A  i_nominal_specify=off  i_nominal_unit=A  i_nominal_value=1  v_specify=off  v_priority=None  v=400 V  v_nominal_specify=off  v_nominal_unit=V  v_nominal_value=1  vc_specify=on  vc_priority=High  vc=48 V  vc_nominal_specify=off  vc_nominal_unit=V  vc_nominal_value=1
  DCL : ee_lib/Passive/Inductor  l=10e-6 H  L_tol=20  enable_L_tol=0  tol_distribution=1  nSigma=4  r=0.1 Ohm  g=1e-9 1/Ohm  enable_operating_limits=0  operating_limit_action=2  max_working_current=1 A  power_rating=1 W  enable_faults=0  fault_action=1  lambdaPercent=50  k_faulted=0.9999  turnsShort=0  openCct=0  groundShort=0  groundShortG=0 1/Ohm  tau_fault=1e-3 s  enable_temporal_fault=0  t_fault=1 s  enable_behavioral_fault=0  max_permissible_voltage=100 V  n_fail_on_voltage=1  max_permissible_current=1 A  t_fail_on_current=1 s  i_L_specify=off  i_L_priority=High  i_L=0 A  i_L_nominal_specify=off  i_L_nominal_unit=A  i_L_nominal_value=1
  Simulink-PS Converter2 : nesl_utility/Simulink-PS Converter  PhysicalDomain=network_engine_domain  SubClassName=ps_input  LeftPortType=input  RightPortType=output  PseudoPeriodic=off  Frequencies=[]  NoiseDistribution=none  NoiseParameters=[]  Unit=1  AffineConversion=off  FilteringAndDerivatives=provide  SimscapeFilterOrder=1  InputFilterTimeConstant=0.001  UdotUserProvided=0
      settings: SourceProductBaseCode=PW,SS
  Subsystem3 : Subsystem
      settings: PortSchema="{\"entries\":[{\"content\":{\"sides\":[{\"content\":{\"connectorIds\":[]},\"type\":\"ConnectorPlacement.EquallySpacedRectSide\",\"uuid\":\"7286f59e-cee0-499d-832c-cf6f33a1b017\"},{\"content\":{\"connectorIds\":[\"Out1\"],\"side\":\"RIGHT\"},\"type\":\"ConnectorPlacement.EquallySpacedRectSide\",\"uuid\":\"6a983281-a6bc-4a57-a5ba-c4da9a8828f4\"},{\"content\":{\"connectorIds\":[\"LConn1\"],\"side\":\"TOP\"},\"type\":\"ConnectorPlacement.EquallySpacedRectSide\",\"uuid\":\"6969f7e7-2dce-4d64-b6f6-e92ef9035b1a\"},{\"content\":{\"connectorIds\":[\"RConn1\"],\"side\":\"BOTTOM\"},\"type\":\"ConnectorPlacement.EquallySpacedRectSide\",\"uuid\":\"8f7d22cd-967a-487e-912d-7270502758f1\"}]},\"type\":\"ConnectorPlacement.EquallySpacedConnector\",\"uuid\":\"05fc616a-5402-4b75-b59e-8cf259d71f3d\"}],\"packageUris\":[\"http://schema.mathworks.com/mf0/Connector/R2020b\"],\"version\":\"1.0\"}"
  DD+ : PMIOPort  Side=Left
  DD- : PMIOPort  Port=2  Side=Left
  Load+ : PMIOPort  Port=3  Side=Right
  Load- : PMIOPort  Port=4  Side=Right
  iLoad48V : Outport
  V48Line : Outport  Port=2
  wires:
  CurrentSensor3/1(iLoad48V) -> iLoad48V/1
  Subsystem3/1(V48Line) -> V48Line/1
  Duty_DCDC/1 -> Simulink-PS Converter2/1
  connections:
  DD+/RConn1 -- Averaged DCDC/LConn2
  CurrentSensor3/RConn1 -- Subsystem3/LConn1 -- Load+/RConn1
  DCL/LConn1 -- Averaged DCDC/RConn1
  DCL/RConn1 -- DCC/LConn1 -- CurrentSensor3/LConn1
  DD-/RConn1 -- Averaged DCDC/LConn3
  DCC/RConn1 -- Averaged DCDC/RConn2 -- Load-/RConn1 -- Subsystem3/RConn1
  Simulink-PS Converter2/RConn1 -- Averaged DCDC/LConn1

== system PlantArch/HVtoMV_DCDC/Subsystem2 ==
  PS-Simulink Converter1 : nesl_utility/PS-Simulink Converter  PhysicalDomain=network_engine_domain  SubClassName=ps_output  LeftPortType=input  RightPortType=output  PseudoPeriodic=off  Frequencies=[]  Unit=inherit  AffineConversion=off
      settings: SourceProductBaseCode=PW,SS
  Voltage Sensor1 : fl_lib/Electrical/Electrical Sensors/Voltage Sensor
  + : PMIOPort  Side=Left
  - : PMIOPort  Port=2  Side=Right
  Vdc : Outport
  wires:
  PS-Simulink Converter1/1 -> Vdc/1  "Vdc"
  connections:
  Voltage Sensor1/RConn2 -- -/RConn1
  Voltage Sensor1/LConn1 -- +/RConn1
  Voltage Sensor1/RConn1 -- PS-Simulink Converter1/LConn1

== system PlantArch/OnbordCharger/CurrentSensor2 ==
  Current Sensor : fl_lib/Electrical/Electrical Sensors/Current Sensor
  PS-Simulink Converter2 : nesl_utility/PS-Simulink Converter  PhysicalDomain=network_engine_domain  SubClassName=ps_output  LeftPortType=input  RightPortType=output  PseudoPeriodic=off  Frequencies=[]  Unit=inherit  AffineConversion=off
      settings: SourceProductBaseCode=PW,SS
  - : PMIOPort  Side=Left
  + : PMIOPort  Port=2  Side=Right
  iDCInv : Outport
  wires:
  PS-Simulink Converter2/1 -> iDCInv/1  "iDCInv"
  connections:
  Current Sensor/RConn2 -- -/RConn1
  PS-Simulink Converter2/LConn1 -- Current Sensor/RConn1
  Current Sensor/LConn1 -- +/RConn1

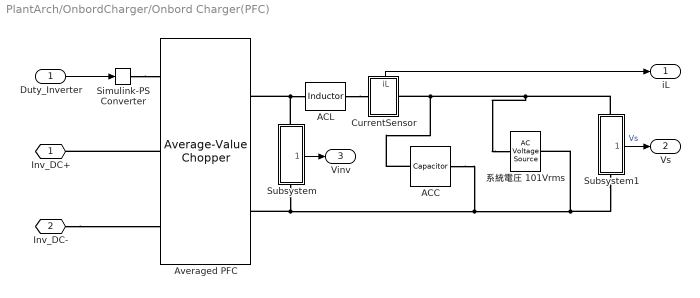
== system PlantArch/OnbordCharger/Onbord Charger(PFC) ==
  Duty_Inverter : Inport
  ACC : ee_lib/Passive/Capacitor  cap_option=0  c=10e-6 F  Cvec=[1e-05, 1e-06] F  Vvec=[0, 10] V  CV_table_symmetry=1  f_vec=[1, 10] kHz  DFext_vec=[.8, 1.2]  C_tol=5  enable_C_tol=0  tol_distribution=1  nSigma=4  r=100e-3 Ohm  g=0 1/Ohm  averaging_period=0 s  enable_operating_limits=0  operating_limit_action=2  max_working_voltage_range=[-25, 25] V  power_rating=1 W  enable_faults=0  fault_action=1  Cscale_faulted=100  R_faulted=1e-3 Ohm  G_faulted=0 1/Ohm  tau_fault=1e-3 s  enable_temporal_fault=0  t_fault=1 s  enable_behavioral_fault=0  max_permissible_voltage_range=[-100, 100] V  t_fail_on_voltage=1 s  i_specify=off  i_priority=None  i=0 A  i_nominal_specify=off  i_nominal_unit=A  i_nominal_value=1  v_specify=off  v_priority=None  v=400 V  v_nominal_specify=off  v_nominal_unit=V  v_nominal_value=1  vc_specify=off  vc_priority=High  vc=48 V  vc_nominal_specify=off  vc_nominal_unit=V  vc_nominal_value=1
  ACL : ee_lib/Passive/Inductor  l=1e-3 H  L_tol=20  enable_L_tol=0  tol_distribution=1  nSigma=4  r=0.1 Ohm  g=1e-9 1/Ohm  enable_operating_limits=0  operating_limit_action=2  max_working_current=1 A  power_rating=1 W  enable_faults=0  fault_action=1  lambdaPercent=50  k_faulted=0.9999  turnsShort=0  openCct=0  groundShort=0  groundShortG=0 1/Ohm  tau_fault=1e-3 s  enable_temporal_fault=0  t_fault=1 s  enable_behavioral_fault=0  max_permissible_voltage=100 V  n_fail_on_voltage=1  max_permissible_current=1 A  t_fail_on_current=1 s  i_L_specify=off  i_L_priority=High  i_L=0 A  i_L_nominal_specify=off  i_L_nominal_unit=A  i_L_nominal_value=1
  Averaged PFC : ee_lib/Semiconductors & Converters/Converters/Average-Value Chopper  chopper_type=5  efficiency_option=1  efficiency_fixed=100  i_vec=[0, 2, 5] A  efficiency_vec=[90, 95, 98]
      settings: SourceProductBaseCode=PS  InternalSimscapePortConfiguration="{\"Bottom\":[],\"Left\":[{\"id\":\"DutyCycle\",\"label\":\"DutyCycle\",\"type\":\"input\"},{\"id\":\"p1\",\"label\":\"1+\",\"type\":\"foundation.electrical.electrical\"},{\"id\":\"n1\",\"label\":\"1-\",\"type\":\"foundation.electrical.electrical\"}],\"Right\":[{\"id\":\"p2\",\"label\":\"2+\",\"type\":\"foundation.electrical.electrical\"},{\"id\":\"n2\",\"label\":\"2-\",\"type\":\"foundation.electrical.electrical\"}],\"Top\":[]}"
  CurrentSensor : Subsystem
      settings: PortSchema="{\"entries\":[{\"content\":{\"sides\":[{\"content\":{\"connectorIds\":[\"LConn1\"]},\"type\":\"ConnectorPlacement.EquallySpacedRectSide\",\"uuid\":\"7286f59e-cee0-499d-832c-cf6f33a1b017\"},{\"content\":{\"connectorIds\":[\"RConn1\"],\"side\":\"RIGHT\"},\"type\":\"ConnectorPlacement.EquallySpacedRectSide\",\"uuid\":\"6a983281-a6bc-4a57-a5ba-c4da9a8828f4\"},{\"content\":{\"connectorIds\":[\"Out1\"],\"side\":\"TOP\"},\"type\":\"ConnectorPlacement.EquallySpacedRectSide\",\"uuid\":\"6969f7e7-2dce-4d64-b6f6-e92ef9035b1a\"}]},\"type\":\"ConnectorPlacement.EquallySpacedConnector\",\"uuid\":\"05fc616a-5402-4b75-b59e-8cf259d71f3d\"}],\"packageUris\":[\"http://schema.mathworks.com/mf0/Connector/R2020b\"],\"version\":\"1.0\"}"
  Simulink-PS Converter : nesl_utility/Simulink-PS Converter  PhysicalDomain=network_engine_domain  SubClassName=ps_input  LeftPortType=input  RightPortType=output  PseudoPeriodic=off  Frequencies=[]  NoiseDistribution=none  NoiseParameters=[]  Unit=1  AffineConversion=off  FilteringAndDerivatives=provide  SimscapeFilterOrder=1  InputFilterTimeConstant=0.001  UdotUserProvided=0
      settings: SourceProductBaseCode=PW,SS
  Subsystem : Subsystem
      settings: PortSchema="{\"entries\":[{\"content\":{\"sides\":[{\"content\":{\"connectorIds\":[]},\"type\":\"ConnectorPlacement.EquallySpacedRectSide\",\"uuid\":\"7286f59e-cee0-499d-832c-cf6f33a1b017\"},{\"content\":{\"connectorIds\":[\"Out1\"],\"side\":\"RIGHT\"},\"type\":\"ConnectorPlacement.EquallySpacedRectSide\",\"uuid\":\"6a983281-a6bc-4a57-a5ba-c4da9a8828f4\"},{\"content\":{\"connectorIds\":[\"LConn1\"],\"side\":\"TOP\"},\"type\":\"ConnectorPlacement.EquallySpacedRectSide\",\"uuid\":\"6969f7e7-2dce-4d64-b6f6-e92ef9035b1a\"},{\"content\":{\"connectorIds\":[\"RConn1\"],\"side\":\"BOTTOM\"},\"type\":\"ConnectorPlacement.EquallySpacedRectSide\",\"uuid\":\"8f7d22cd-967a-487e-912d-7270502758f1\"}]},\"type\":\"ConnectorPlacement.EquallySpacedConnector\",\"uuid\":\"05fc616a-5402-4b75-b59e-8cf259d71f3d\"}],\"packageUris\":[\"http://schema.mathworks.com/mf0/Connector/R2020b\"],\"version\":\"1.0\"}"
  Subsystem1 : Subsystem
      settings: PortSchema="{\"entries\":[{\"content\":{\"sides\":[{\"content\":{\"connectorIds\":[]},\"type\":\"ConnectorPlacement.EquallySpacedRectSide\",\"uuid\":\"7286f59e-cee0-499d-832c-cf6f33a1b017\"},{\"content\":{\"connectorIds\":[\"Out1\"],\"side\":\"RIGHT\"},\"type\":\"ConnectorPlacement.EquallySpacedRectSide\",\"uuid\":\"6a983281-a6bc-4a57-a5ba-c4da9a8828f4\"},{\"content\":{\"connectorIds\":[\"LConn1\"],\"side\":\"TOP\"},\"type\":\"ConnectorPlacement.EquallySpacedRectSide\",\"uuid\":\"6969f7e7-2dce-4d64-b6f6-e92ef9035b1a\"},{\"content\":{\"connectorIds\":[\"RConn1\"],\"side\":\"BOTTOM\"},\"type\":\"ConnectorPlacement.EquallySpacedRectSide\",\"uuid\":\"8f7d22cd-967a-487e-912d-7270502758f1\"}]},\"type\":\"ConnectorPlacement.EquallySpacedConnector\",\"uuid\":\"05fc616a-5402-4b75-b59e-8cf259d71f3d\"}],\"packageUris\":[\"http://schema.mathworks.com/mf0/Connector/R2020b\"],\"version\":\"1.0\"}"
  系統電圧 101Vrms : fl_lib/Electrical/Electrical Sources/AC Voltage Source  amp=101*1.414 V  shift=0 deg  frequency=60 Hz  omega=0 rad/s
  Inv_DC+ : PMIOPort  Side=Left
  Inv_DC- : PMIOPort  Port=2  Side=Left
  iL : Outport
  Vs : Outport  Port=2
  Vinv : Outport  Port=3
  wires:
  Subsystem1/1(Vs) -> Vs/1  "Vs"
  Subsystem/1(Vinv) -> Vinv/1
  CurrentSensor/1(iL) -> iL/1
  Duty_Inverter/1 -> Simulink-PS Converter/1
  connections:
  Averaged PFC/LConn2 -- Inv_DC+/RConn1
  Inv_DC-/RConn1 -- Averaged PFC/LConn3
  Simulink-PS Converter/RConn1 -- Averaged PFC/LConn1
  系統電圧 101Vrms/LConn1 -- CurrentSensor/RConn1 -- ACC/LConn1 -- Subsystem1/LConn1
  ACL/LConn1 -- Averaged PFC/RConn1 -- Subsystem/LConn1
  系統電圧 101Vrms/RConn1 -- Subsystem/RConn1 -- Averaged PFC/RConn2 -- ACC/RConn1 -- Subsystem1/RConn1
  ACL/RConn1 -- CurrentSensor/LConn1

== system PlantArch/OnbordCharger/Subsystem2 ==
  PS-Simulink Converter1 : nesl_utility/PS-Simulink Converter  PhysicalDomain=network_engine_domain  SubClassName=ps_output  LeftPortType=input  RightPortType=output  PseudoPeriodic=off  Frequencies=[]  Unit=inherit  AffineConversion=off
      settings: SourceProductBaseCode=PW,SS
  Voltage Sensor1 : fl_lib/Electrical/Electrical Sensors/Voltage Sensor
  + : PMIOPort  Side=Left
  - : PMIOPort  Port=2  Side=Right
  Vdc : Outport
  wires:
  PS-Simulink Converter1/1 -> Vdc/1  "Vdc"
  connections:
  Voltage Sensor1/RConn2 -- -/RConn1
  Voltage Sensor1/LConn1 -- +/RConn1
  Voltage Sensor1/RConn1 -- PS-Simulink Converter1/LConn1

== system PlantArch/HVtoMV_DCDC/High to MiddlleVoltage DCDC Converter/CurrentSensor3 ==
  Current Sensor : fl_lib/Electrical/Electrical Sensors/Current Sensor
  PS-Simulink Converter2 : nesl_utility/PS-Simulink Converter  PhysicalDomain=network_engine_domain  SubClassName=ps_output  LeftPortType=input  RightPortType=output  PseudoPeriodic=off  Frequencies=[]  Unit=inherit  AffineConversion=off
      settings: SourceProductBaseCode=PW,SS
  + : PMIOPort  Side=Left
  - : PMIOPort  Port=2  Side=Right
  iLoad48V : Outport
  wires:
  PS-Simulink Converter2/1 -> iLoad48V/1  "iLoad48V"
  connections:
  Current Sensor/RConn2 -- -/RConn1
  PS-Simulink Converter2/LConn1 -- Current Sensor/RConn1
  Current Sensor/LConn1 -- +/RConn1

== system PlantArch/HVtoMV_DCDC/High to MiddlleVoltage DCDC Converter/Subsystem3 ==
  PS-Simulink Converter1 : nesl_utility/PS-Simulink Converter  PhysicalDomain=network_engine_domain  SubClassName=ps_output  LeftPortType=input  RightPortType=output  PseudoPeriodic=off  Frequencies=[]  Unit=inherit  AffineConversion=off
      settings: SourceProductBaseCode=PW,SS
  Voltage Sensor1 : fl_lib/Electrical/Electrical Sensors/Voltage Sensor
  + : PMIOPort  Side=Left
  - : PMIOPort  Port=2  Side=Right
  V48Line : Outport
  wires:
  PS-Simulink Converter1/1 -> V48Line/1  "V48Line"
  connections:
  Voltage Sensor1/RConn2 -- -/RConn1
  Voltage Sensor1/LConn1 -- +/RConn1
  Voltage Sensor1/RConn1 -- PS-Simulink Converter1/LConn1

== system PlantArch/OnbordCharger/Onbord Charger(PFC)/CurrentSensor ==
  Current Sensor : fl_lib/Electrical/Electrical Sensors/Current Sensor
  PS-Simulink Converter2 : nesl_utility/PS-Simulink Converter  PhysicalDomain=network_engine_domain  SubClassName=ps_output  LeftPortType=input  RightPortType=output  PseudoPeriodic=off  Frequencies=[]  Unit=inherit  AffineConversion=off
      settings: SourceProductBaseCode=PW,SS
  + : PMIOPort  Side=Left
  - : PMIOPort  Port=2  Side=Right
  iL : Outport
  wires:
  PS-Simulink Converter2/1 -> iL/1  "iL"
  connections:
  Current Sensor/RConn2 -- -/RConn1
  PS-Simulink Converter2/LConn1 -- Current Sensor/RConn1
  Current Sensor/LConn1 -- +/RConn1

== system PlantArch/OnbordCharger/Onbord Charger(PFC)/Subsystem ==
  PS-Simulink Converter1 : nesl_utility/PS-Simulink Converter  PhysicalDomain=network_engine_domain  SubClassName=ps_output  LeftPortType=input  RightPortType=output  PseudoPeriodic=off  Frequencies=[]  Unit=inherit  AffineConversion=off
      settings: SourceProductBaseCode=PW,SS
  Voltage Sensor1 : fl_lib/Electrical/Electrical Sensors/Voltage Sensor
  + : PMIOPort  Side=Left
  - : PMIOPort  Port=2  Side=Right
  Vinv : Outport
  wires:
  PS-Simulink Converter1/1 -> Vinv/1  "Vinv"
  connections:
  Voltage Sensor1/RConn2 -- -/RConn1
  Voltage Sensor1/LConn1 -- +/RConn1
  Voltage Sensor1/RConn1 -- PS-Simulink Converter1/LConn1

== system PlantArch/OnbordCharger/Onbord Charger(PFC)/Subsystem1 ==
  PS-Simulink Converter1 : nesl_utility/PS-Simulink Converter  PhysicalDomain=network_engine_domain  SubClassName=ps_output  LeftPortType=input  RightPortType=output  PseudoPeriodic=off  Frequencies=[]  Unit=inherit  AffineConversion=off
      settings: SourceProductBaseCode=PW,SS
  Voltage Sensor1 : fl_lib/Electrical/Electrical Sensors/Voltage Sensor
  + : PMIOPort  Side=Left
  - : PMIOPort  Port=2  Side=Right
  Vs : Outport
  wires:
  PS-Simulink Converter1/1 -> Vs/1  "Vs"
  connections:
  Voltage Sensor1/RConn2 -- -/RConn1
  Voltage Sensor1/LConn1 -- +/RConn1
  Voltage Sensor1/RConn1 -- PS-Simulink Converter1/LConn1
